simulink model "Attitude_control_RW_20b"  (R2022a)
settings: Solver=VariableStepAuto  StartTime=0.0  StopTime=100  FixedStep=0.0001  RelTol=1e-3
values from neighbouring files (symbols this model uses):
  D = 9.4e-5*Kt    (= 4.7e-06)    [motor_parameter.m]
  J = 1.94e-4*Kt    (= 9.7e-06)    [motor_parameter.m]
  kii = (J*(-Kt^2+kpo*R)*wn^2)/(Kt*(D^2+kpo^2+J^2*wn^2-2*J*kpo*wn*zeta+2*D*(kpo-J*wn*zeta)))    (= 0.394297267374)    [motor_parameter.m]
  kpi = -(D^2*R+J^2*R*wn^2+kpo*(Kt^2-2*J*R*wn*zeta)+D*(Kt^2+R*(kpo-2*J*wn*zeta))/(Kt*(D^2+kpo^2+J^2*wn^2-2*J*kpo*wn*zeta+2*D*(kpo-J*wn*zeta))))    (= 0.0794485412984)    [motor_parameter.m]
  kpo = 10    [motor_parameter.m]
  Kt = 0.05    [motor_parameter.m]
  L = 0.001    [motor_parameter.m]
  R = 14.3    [motor_parameter.m]
  Tc = 0.053*Kt    (= 0.00265)    [motor_parameter.m]
undefined symbols (not defined in the file or in its folder): b, Is, kk, Km, Q, q_init, Rgyro, Rstr, rw_Inertia, rw_SensorToBody, Ts, unit7, w0, w_dot_init, w_init, wRW_init
libraries: simulink_extras x13, sharedtransform x12, simulink x5, slpidlib x3, aerolibutil x2, sharedTrackingLibrary x1
(part 1 of 2)
settings Model: Creator=sokserey  LastModifiedBy=LabPC
settings SolverCC: ZeroCrossAlgorithm=Adaptive  AlgebraicLoopSolver=TrustRegion
settings DebuggingCC: IgnoredZcDiagnostic=none  UnconnectedInputMsg=warning  UnconnectedOutputMsg=warning  UnconnectedLineMsg=warning
settings RTWCC: DLArmComputeVersion=19.05

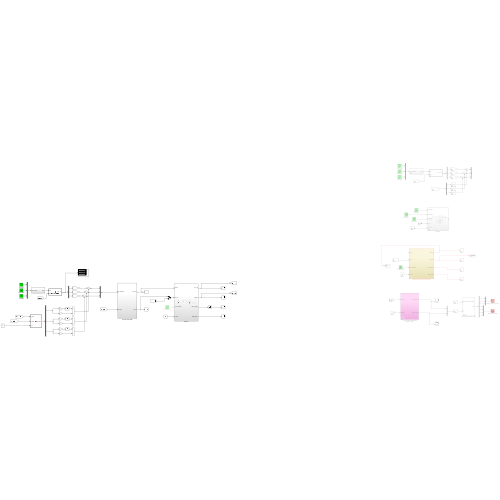
[thumbnail: Simulink's stored preview of the top-level diagram]
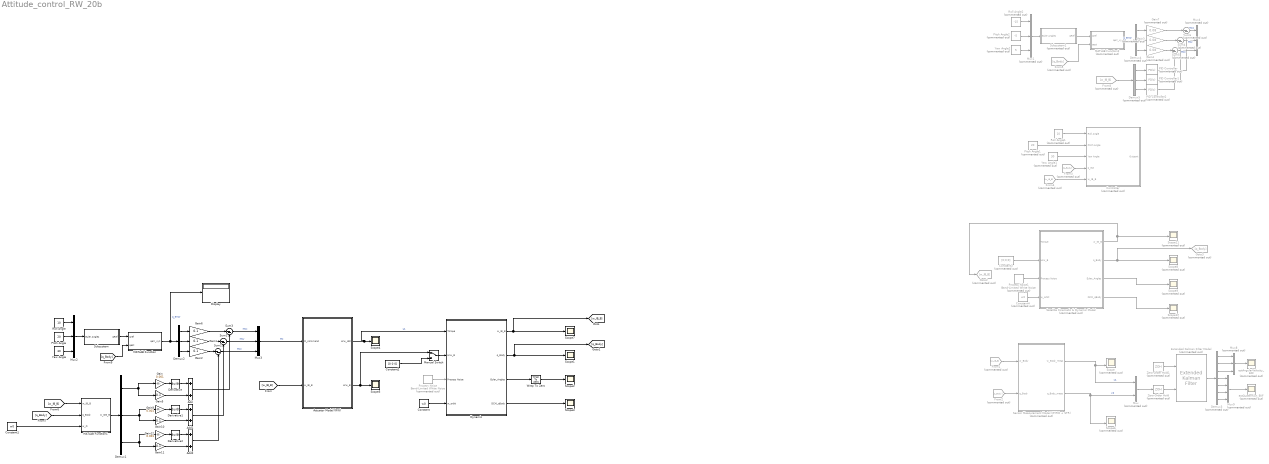
== system Attitude_control_RW_20b ==
  Actuator Model (RW) : Subsystem
  Add : Sum
  Add1 : Sum
  Add2 : Sum
  Constant : Constant  Value=w0
  Constant1 : Constant  Value=w0
  Constant2 : Constant  Value=[0 0 0]
  Constant3 : Constant  Commented=on  Value=[0;0;0]
  Constant4 : Constant  Commented=on  Value=w0
  Controller : Subsystem  Commented=on
  Demux1 : Demux  Outputs=3
  Demux2 : Demux  Outputs=3
  Demux3 : Demux  Commented=on  Outputs=7
  Demux4 : Demux  Commented=on  Outputs=3
  Demux5 : Demux  Commented=on  Outputs=3
  Derivative : Derivative
  Derivative1 : Derivative
  Derivative2 : Derivative
  Display : Display
  Dynamic : Subsystem
  "Extended Kalman Filter Model " : sharedTrackingLibrary/Extended Kalman Filter  Commented=on  StateTransitionFcn=dynamicFunctions2  HasStateTransitionJacobianFcn=off  HasAdditiveProcessNoise=Additive  ProcessNoise=diag(unit7)*Q  HasTimeVaryingProcessNoise=off  HasStateTransitionFcnExtraArgument=1  InitialState=[w_init; q_init]  InitialStateCovariance=1e-6  MeasurementFcn1=measurementFunction2  HasMeasurementJacobianFcn1=off  HasMeasurementEnablePort1=off  HasAdditiveMeasurementNoise1=Additive  MeasurementNoise1=Rconf4  HasTimeVaryingMeasurementNoise1=off  HasMeasurementFcnExtraArgument1=0  HasMeasurementWrapping1=off  MeasurementFcn2=myMeasurementFcn  HasMeasurementJacobianFcn2=off  HasMeasurementEnablePort2=off  HasAdditiveMeasurementNoise2=Additive  MeasurementNoise2=1  HasTimeVaryingMeasurementNoise2=off  HasMeasurementFcnExtraArgument2=0  HasMeasurementWrapping2=off  MeasurementFcn3=myMeasurementFcn  HasMeasurementJacobianFcn3=off  HasMeasurementEnablePort3=off  HasAdditiveMeasurementNoise3=Additive  MeasurementNoise3=1  HasTimeVaryingMeasurementNoise3=off  HasMeasurementFcnExtraArgument3=0  HasMeasurementWrapping3=off  MeasurementFcn4=myMeasurementFcn  HasMeasurementJacobianFcn4=off  HasMeasurementEnablePort4=off  HasAdditiveMeasurementNoise4=Additive  MeasurementNoise4=1  HasTimeVaryingMeasurementNoise4=off  HasMeasurementFcnExtraArgument4=0  HasMeasurementWrapping4=off  MeasurementFcn5=myMeasurementFcn  HasMeasurementJacobianFcn5=off  HasMeasurementEnablePort5=off  HasAdditiveMeasurementNoise5=Additive  MeasurementNoise5=1  HasTimeVaryingMeasurementNoise5=off  HasMeasurementFcnExtraArgument5=0  HasMeasurementWrapping5=off  EnableMultirate=off  StateTransitionFcnSampleTime=1  MeasurementFcn1SampleTime=1  MeasurementFcn2SampleTime=1  MeasurementFcn3SampleTime=1  MeasurementFcn4SampleTime=1  MeasurementFcn5SampleTime=1  UseCurrentEstimator=on  OutputStateCovariance=off  DataType=double  SampleTime=Ts  NumberOfMeasurements=1
      settings: SourceProductBaseCode=TF,AE,PW,CT,DR,ID,LP,NV,AR,RO,RR,UV,VE
  From1 : From  Commented=on  GotoTag=w_IB_B
  From2 : From  Commented=on  GotoTag=q_Body
  From3 : From  Commented=on  GotoTag=q_Body
  From4 : From  Commented=on  GotoTag=w_IB_B
  From5 : From  Commented=on  GotoTag=q_Body
  From8 : From  Commented=on  GotoTag=w_IB_B
  Gain : Gain  Gain=0.001
  Gain{1..2,5..6,10..11} (6 alike) : Gain  Gain=0.1
  Gain12 : Gain  Gain=0.001
  Gain3 : Gain  Commented=on  Gain=0.08
  Gain4 : Gain  Commented=on  Gain=0.08
  Gain7 : Gain  Commented=on  Gain=0.08
  Gain9 : Gain  Gain=0.001
  Goto2 : Goto  Commented=on  GotoTag=w_IB_B
  Goto3 : Goto  Commented=on  GotoTag=q_Body
  MATLAB Function : MATLAB Function  TreatAsAtomicUnit=on
  MATLAB Function1 : MATLAB Function  TreatAsAtomicUnit=on
  MATLAB Function2 : MATLAB Function  Commented=on  TreatAsAtomicUnit=on
  Manual Switch : ManualSwitch
  Mux : Mux  Commented=on  Inputs=2
  Mux1 : Mux  Commented=on  Inputs=3
  Mux2 : Mux  Inputs=3
  Mux3 : Mux  Inputs=3
  Mux4 : Mux  Commented=on  Inputs=3
  Mux8 : Mux  Commented=on  Inputs=3
  Mux9 : Mux  Commented=on
  PID Controller : slpidlib/PID Controller  Commented=on  Controller=PD  Form=Parallel  TimeDomain=Continuous-time  UseExternalTs=off  SampleTime=-1  IntegratorMethod=Forward Euler  FilterMethod=Forward Euler  ControllerParametersSource=internal  P=1  I=2  UseKiTs=off  D=2  N=100  UseFilter=on  TunerSelectOption=Transfer Function Based (PID Tuner App)  InitialConditionSource=internal  InitialConditionForIntegrator=0  InitialConditionForFilter=0  DifferentiatorICPrevScaledInput=0  ExternalReset=none  TrackingMode=off  Kt=1  LimitOutput=off  SatLimitsSource=internal  UpperSaturationLimit=inf  LowerSaturationLimit=-inf  LinearizeAsGain=on  AntiWindupMode=none  Kb=1  POutMin=[]  POutMax=[]  IOutMin=[]  IOutMax=[]  DOutMin=[]  DOutMax=[]  NOutMin=[]  NOutMax=[]  SumOutMin=[]  SumOutMax=[]  SaturationOutMin=[]  SaturationOutMax=[]  PParamMin=[]  PParamMax=[]  IParamMin=[]  IParamMax=[]  DParamMin=[]  DParamMax=[]  NParamMin=[]  NParamMax=[]  KbParamMin=[]  KbParamMax=[]  KtParamMin=[]  KtParamMax=[]  KbOutMin=[]  KbOutMax=[]  KtOutMin=[]  KtOutMax=[]  IntegratorOutMin=[]  IntegratorOutMax=[]  FilterOutMin=[]  FilterOutMax=[]  SumI1OutMin=[]  SumI1OutMax=[]  SumI2OutMin=[]  SumI2OutMax=[]  SumI3OutMin=[]  SumI3OutMax=[]  SumI4OutMin=[]  SumI4OutMax=[]  SumDOutMin=[]  SumDOutMax=[]  DifferentiatorOutMin=[]  DifferentiatorOutMax=[]  FilterDiffOutCoefMin=[]  FilterDiffOutCoefMax=[]  ReciprocalOutMin=[]  ReciprocalOutMax=[]  SumDenOutMin=[]  SumDenOutMax=[]  SumNumOutMin=[]  SumNumOutMax=[]  DivideOutMin=[]  DivideOutMax=[]  UdiffTsProdOutMin=[]  UdiffTsProdOutMax=[]  NTsProdOutMin=[]  NTsProdOutMax=[]  UintegralTsProdOutMin=[]  UintegralTsProdOutMax=[]  UngainTsProdOutMin=[]  UngainTsProdOutMax=[]  IntegratorContinuousStateAttributes=''  IntegratorStateMustResolveToSignalObject=off  IntegratorRTWStateStorageClass=Auto  FilterContinuousStateAttributes=''  FilterStateMustResolveToSignalObject=off  FilterRTWStateStorageClass=Auto  ParallelPVariant=InternalParameters  IdealPVariant=Disabled  IVariant=Disabled  DVariant=InternalParameters  IntegratorVariant=Disabled  SatVariant=Disabled  AWVariant=Disabled  PCopyVariant=Disabled  TRVariant=Disabled  FdbkBlocksVariant=Forward  IdealPFdbkVariant=Disabled  SatFdbkVariant=Disabled  DerivativeFilterVariant=ContFilter  NVariant=InternalParameters  NCopyVariant=Disabled  FilterICVariant=InternalICsFilter  IntegratorICVariant=Disabled  ExternalResetVariant=Disabled  TRSumVariant=Passthrough  SumFdbkVariant=Disabled  SumVariant=Sum_PD  TsampFilterVariant=InternalTs  TsampNgainVariant=Passthrough  TsampIntegralVariant=Disabled_SignalSpec  ExternalSaturationOutDataTypeStr=Inherit: Same as second input  aMode=0
  PID Controller1 : slpidlib/PID Controller  Commented=on  Controller=PD  Form=Parallel  TimeDomain=Continuous-time  UseExternalTs=off  SampleTime=-1  IntegratorMethod=Forward Euler  FilterMethod=Forward Euler  ControllerParametersSource=internal  P=1  I=2  UseKiTs=off  D=2  N=100  UseFilter=on  TunerSelectOption=Transfer Function Based (PID Tuner App)  InitialConditionSource=internal  InitialConditionForIntegrator=0  InitialConditionForFilter=0  DifferentiatorICPrevScaledInput=0  ExternalReset=none  TrackingMode=off  Kt=1  LimitOutput=off  SatLimitsSource=internal  UpperSaturationLimit=inf  LowerSaturationLimit=-inf  LinearizeAsGain=on  AntiWindupMode=none  Kb=1  POutMin=[]  POutMax=[]  IOutMin=[]  IOutMax=[]  DOutMin=[]  DOutMax=[]  NOutMin=[]  NOutMax=[]  SumOutMin=[]  SumOutMax=[]  SaturationOutMin=[]  SaturationOutMax=[]  PParamMin=[]  PParamMax=[]  IParamMin=[]  IParamMax=[]  DParamMin=[]  DParamMax=[]  NParamMin=[]  NParamMax=[]  KbParamMin=[]  KbParamMax=[]  KtParamMin=[]  KtParamMax=[]  KbOutMin=[]  KbOutMax=[]  KtOutMin=[]  KtOutMax=[]  IntegratorOutMin=[]  IntegratorOutMax=[]  FilterOutMin=[]  FilterOutMax=[]  SumI1OutMin=[]  SumI1OutMax=[]  SumI2OutMin=[]  SumI2OutMax=[]  SumI3OutMin=[]  SumI3OutMax=[]  SumI4OutMin=[]  SumI4OutMax=[]  SumDOutMin=[]  SumDOutMax=[]  DifferentiatorOutMin=[]  DifferentiatorOutMax=[]  FilterDiffOutCoefMin=[]  FilterDiffOutCoefMax=[]  ReciprocalOutMin=[]  ReciprocalOutMax=[]  SumDenOutMin=[]  SumDenOutMax=[]  SumNumOutMin=[]  SumNumOutMax=[]  DivideOutMin=[]  DivideOutMax=[]  UdiffTsProdOutMin=[]  UdiffTsProdOutMax=[]  NTsProdOutMin=[]  NTsProdOutMax=[]  UintegralTsProdOutMin=[]  UintegralTsProdOutMax=[]  UngainTsProdOutMin=[]  UngainTsProdOutMax=[]  IntegratorContinuousStateAttributes=''  IntegratorStateMustResolveToSignalObject=off  IntegratorRTWStateStorageClass=Auto  FilterContinuousStateAttributes=''  FilterStateMustResolveToSignalObject=off  FilterRTWStateStorageClass=Auto  ParallelPVariant=InternalParameters  IdealPVariant=Disabled  IVariant=Disabled  DVariant=InternalParameters  IntegratorVariant=Disabled  SatVariant=Disabled  AWVariant=Disabled  PCopyVariant=Disabled  TRVariant=Disabled  FdbkBlocksVariant=Forward  IdealPFdbkVariant=Disabled  SatFdbkVariant=Disabled  DerivativeFilterVariant=ContFilter  NVariant=InternalParameters  NCopyVariant=Disabled  FilterICVariant=InternalICsFilter  IntegratorICVariant=Disabled  ExternalResetVariant=Disabled  TRSumVariant=Passthrough  SumFdbkVariant=Disabled  SumVariant=Sum_PD  TsampFilterVariant=InternalTs  TsampNgainVariant=Passthrough  TsampIntegralVariant=Disabled_SignalSpec  ExternalSaturationOutDataTypeStr=Inherit: Same as second input  aMode=0
  PID Controller2 : slpidlib/PID Controller  Commented=on  Controller=PD  Form=Parallel  TimeDomain=Continuous-time  UseExternalTs=off  SampleTime=-1  IntegratorMethod=Forward Euler  FilterMethod=Forward Euler  ControllerParametersSource=internal  P=1  I=2  UseKiTs=off  D=2  N=100  UseFilter=on  TunerSelectOption=Transfer Function Based (PID Tuner App)  InitialConditionSource=internal  InitialConditionForIntegrator=0  InitialConditionForFilter=0  DifferentiatorICPrevScaledInput=0  ExternalReset=none  TrackingMode=off  Kt=1  LimitOutput=off  SatLimitsSource=internal  UpperSaturationLimit=inf  LowerSaturationLimit=-inf  LinearizeAsGain=on  AntiWindupMode=none  Kb=1  POutMin=[]  POutMax=[]  IOutMin=[]  IOutMax=[]  DOutMin=[]  DOutMax=[]  NOutMin=[]  NOutMax=[]  SumOutMin=[]  SumOutMax=[]  SaturationOutMin=[]  SaturationOutMax=[]  PParamMin=[]  PParamMax=[]  IParamMin=[]  IParamMax=[]  DParamMin=[]  DParamMax=[]  NParamMin=[]  NParamMax=[]  KbParamMin=[]  KbParamMax=[]  KtParamMin=[]  KtParamMax=[]  KbOutMin=[]  KbOutMax=[]  KtOutMin=[]  KtOutMax=[]  IntegratorOutMin=[]  IntegratorOutMax=[]  FilterOutMin=[]  FilterOutMax=[]  SumI1OutMin=[]  SumI1OutMax=[]  SumI2OutMin=[]  SumI2OutMax=[]  SumI3OutMin=[]  SumI3OutMax=[]  SumI4OutMin=[]  SumI4OutMax=[]  SumDOutMin=[]  SumDOutMax=[]  DifferentiatorOutMin=[]  DifferentiatorOutMax=[]  FilterDiffOutCoefMin=[]  FilterDiffOutCoefMax=[]  ReciprocalOutMin=[]  ReciprocalOutMax=[]  SumDenOutMin=[]  SumDenOutMax=[]  SumNumOutMin=[]  SumNumOutMax=[]  DivideOutMin=[]  DivideOutMax=[]  UdiffTsProdOutMin=[]  UdiffTsProdOutMax=[]  NTsProdOutMin=[]  NTsProdOutMax=[]  UintegralTsProdOutMin=[]  UintegralTsProdOutMax=[]  UngainTsProdOutMin=[]  UngainTsProdOutMax=[]  IntegratorContinuousStateAttributes=''  IntegratorStateMustResolveToSignalObject=off  IntegratorRTWStateStorageClass=Auto  FilterContinuousStateAttributes=''  FilterStateMustResolveToSignalObject=off  FilterRTWStateStorageClass=Auto  ParallelPVariant=InternalParameters  IdealPVariant=Disabled  IVariant=Disabled  DVariant=InternalParameters  IntegratorVariant=Disabled  SatVariant=Disabled  AWVariant=Disabled  PCopyVariant=Disabled  TRVariant=Disabled  FdbkBlocksVariant=Forward  IdealPFdbkVariant=Disabled  SatFdbkVariant=Disabled  DerivativeFilterVariant=ContFilter  NVariant=InternalParameters  NCopyVariant=Disabled  FilterICVariant=InternalICsFilter  IntegratorICVariant=Disabled  ExternalResetVariant=Disabled  TRSumVariant=Passthrough  SumFdbkVariant=Disabled  SumVariant=Sum_PD  TsampFilterVariant=InternalTs  TsampNgainVariant=Passthrough  TsampIntegralVariant=Disabled_SignalSpec  ExternalSaturationOutDataTypeStr=Inherit: Same as second input  aMode=0
  Pitch Angle : Constant  Value=20
  Pitch Angle1 : Constant  Commented=on  Value=20
  Pitch Angle2 : Constant  Commented=on  Value=-5
  Process Noise : simulink/Sources/Band-Limited White Noise  Commented=on  Cov=Q*Ts  Ts=Ts  seed=[23341]
  Process Noise1 : simulink/Sources/Band-Limited White Noise  Commented=on  Cov=Q*Ts  Ts=Ts  seed=[23341]
  Roll Angle : Constant  Value=10
  Roll Angle1 : Constant  Commented=on  Value=10
  Roll Angle2 : Constant  Commented=on  Value=-15
  Satellite Kinematic & Dynamic Model : Subsystem  Commented=on
  Scope : Scope  Commented=on  NumInputPorts=2
  Scope{1..5,7} (6 alike) : Scope
  Scope{8..11} (4 alike) : Scope  Commented=on
  Scope6 : Scope  Commented=on  NumInputPorts=2
  Sensor Measurement Model (GYRO + STR) : Subsystem  Commented=on
  Subsystem : Subsystem
  Subsystem1 : Subsystem  Commented=on
  Sum1 : Sum  Inputs=|--
  Sum2 : Sum  Inputs=|--
  Sum3 : Sum  Inputs=|--
  Sum4 : Sum  Commented=on  Inputs=|--
  Sum5 : Sum  Commented=on  Inputs=|--
  Sum6 : Sum  Commented=on  Inputs=|--
  Wrap To Zero : simulink/Discontinuities/Wrap To Zero  Threshold=360
      settings: SourceProductBaseCode=SL
  Yaw Angle : Constant  Value=30
  Yaw Angle1 : Constant  Commented=on  Value=30
  Yaw Angle2 : Constant  Commented=on  Value=5
  Zero-Order Hold : ZeroOrderHold  Commented=on  SampleTime=Ts
  Zero-Order Hold1 : ZeroOrderHold  Commented=on  SampleTime=Ts
  estAngularVelocity_EKF : Scope  Commented=on
  "estQuaternion_EKF " : Scope  Commented=on
  wires:
  Process Noise/1 -> Dynamic/3("Process Noise ")
  Constant/1 -> Dynamic/4(w_orbit)
  Dynamic/2(q_Body) -> [q_Body], Scope1/1
  Dynamic/3(Euler_Angles) -> Wrap To Zero/1
  Dynamic/4(DCM_qBody) -> Scope3/1
  Zero-Order Hold1/1 -> "Extended Kalman Filter Model "/1
  Demux3/2 -> Mux8/2
  Demux3/3 -> Mux8/3
  Demux3/6 -> Mux9/3
  Demux3/4 -> Mux9/1
  Mux9/1 -> "estQuaternion_EKF "/1
  Demux3/5 -> Mux9/2
  "Extended Kalman Filter Model "/1 -> Demux3/1
  Demux3/1 -> Mux8/1
  Zero-Order Hold/1 -> "Extended Kalman Filter Model "/2
  [w_IB_B] -> Actuator Model (RW)/2(w_IB_B)
  Actuator Model (RW)/1("Hrw_dot ") -> Dynamic/1(Torque), Scope4/1  "u1"
  From1/1 -> Sensor Measurement Model (GYRO + STR)/1(w_Body)
  Sensor Measurement Model (GYRO + STR)/1(w_Body_meas) -> Mux/1, Scope/2  "y1"
  From2/1 -> Sensor Measurement Model (GYRO + STR)/2(q_Body)
  Sensor Measurement Model (GYRO + STR)/2(q_Body_meas) -> Scope6/2, Mux/2  "y2"
  Mux/1 -> Zero-Order Hold/1
  Roll Angle/1 -> Mux2/1
  Sum1/1 -> Mux3/2  "Mcy"
  MATLAB Function/1(qerr_xyz) -> Display/1, Demux2/1  "q_error"
  Sum3/1 -> Mux3/1  "Mcx"
  Gain2/1 -> Sum2/1
  Sum2/1 -> Mux3/3  "Mcz"
  Demux2/2 -> Gain1/1
  Demux2/1 -> Gain6/1
  Gain6/1 -> Sum3/1
  Yaw Angle/1 -> Mux2/3
  Subsystem/1(qRef) -> MATLAB Function/1(qref)
  Gain1/1 -> Sum1/1
  Pitch Angle/1 -> Mux2/2
  Mux2/1 -> Subsystem/1(Euler Angles)
  Demux2/3 -> Gain2/1
  Mux8/1 -> estAngularVelocity_EKF/1
  Demux3/7 -> Mux9/4
  Dynamic/1(w_IB_B) -> [w_IB_B], Scope7/1
  Roll Angle1/1 -> Controller/1("Roll Angle ")
  Pitch Angle1/1 -> Controller/2("Pitch Angle ")
  Yaw Angle1/1 -> Controller/3("Yaw Angle ")
  Actuator Model (RW)/2(Hrw_B) -> Manual Switch/1, Scope5/1
  From3/1 -> Controller/4(q_est)
  From4/1 -> Controller/5(w_IB_B)
  Derivative/1 -> Add/1
  Gain5/1 -> Add/2
  Gain9/1 -> Derivative1/1
  Gain10/1 -> Add1/2
  Gain11/1 -> Add2/2
  Derivative1/1 -> Add1/1
  Demux1/3 -> Gain12/1, Gain11/1
  Gain/1 -> Derivative/1
  Derivative2/1 -> Add2/1
  Demux1/1 -> Gain/1, Gain5/1
  Demux1/2 -> Gain9/1, Gain10/1
  Gain12/1 -> Derivative2/1
  [w_IB_B] -> MATLAB Function1/1(w_IB_B)
  [q_Body] -> MATLAB Function1/2(q_Body)
  Constant1/1 -> MATLAB Function1/3(w_O)
  MATLAB Function1/1(w_OB_B) -> Demux1/1
  Manual Switch/1 -> Dynamic/2(Hrw_B)
  Constant2/1 -> Manual Switch/2
  Demux4/2 -> Gain3/1
  Sum6/1 -> Mux4/1  "Mcx"
  Sum5/1 -> Mux4/3  "Mcz"
  Gain7/1 -> Sum6/1
  PID Controller1/1 -> Sum4/2
  PID Controller2/1 -> Sum5/2
  Gain4/1 -> Sum5/1
  Sum4/1 -> Mux4/2  "Mcy"
  Demux5/3 -> PID Controller2/1
  PID Controller/1 -> Sum6/2
  Subsystem1/1(qRef) -> MATLAB Function2/1(qref)
  Demux5/1 -> PID Controller/1
  Demux5/2 -> PID Controller1/1
  Demux4/3 -> Gain4/1
  MATLAB Function2/1(qerr_xyz) -> Demux4/1  "q_error"
  Demux4/1 -> Gain7/1
  Pitch Angle2/1 -> Mux1/2
  Gain3/1 -> Sum4/1
  Yaw Angle2/1 -> Mux1/3
  Roll Angle2/1 -> Mux1/1
  Mux1/1 -> Subsystem1/1(Euler Angles)
  From8/1 -> Demux5/1
  From5/1 -> MATLAB Function2/2(qest)
  Constant3/1 -> Satellite Kinematic & Dynamic Model/2(Hrw_B)
  Process Noise1/1 -> Satellite Kinematic & Dynamic Model/3("Process Noise ")
  Constant4/1 -> Satellite Kinematic & Dynamic Model/4(w_orbit)
  Satellite Kinematic & Dynamic Model/1(w_IB_B) -> Scope11/1, Goto2/1
  Satellite Kinematic & Dynamic Model/4(DCM_qBody) -> Scope10/1
  Satellite Kinematic & Dynamic Model/3(Euler_Angles) -> Scope9/1
  Satellite Kinematic & Dynamic Model/2(q_Body) -> Scope8/1, Goto3/1
  Add/1 -> Sum3/2
  Add1/1 -> Sum1/2
  Add2/1 -> Sum2/2
  [q_Body] -> MATLAB Function/2(qest)
  Mux3/1 -> Actuator Model (RW)/1("M_command ")  "Mc"
  Wrap To Zero/1 -> Scope2/1

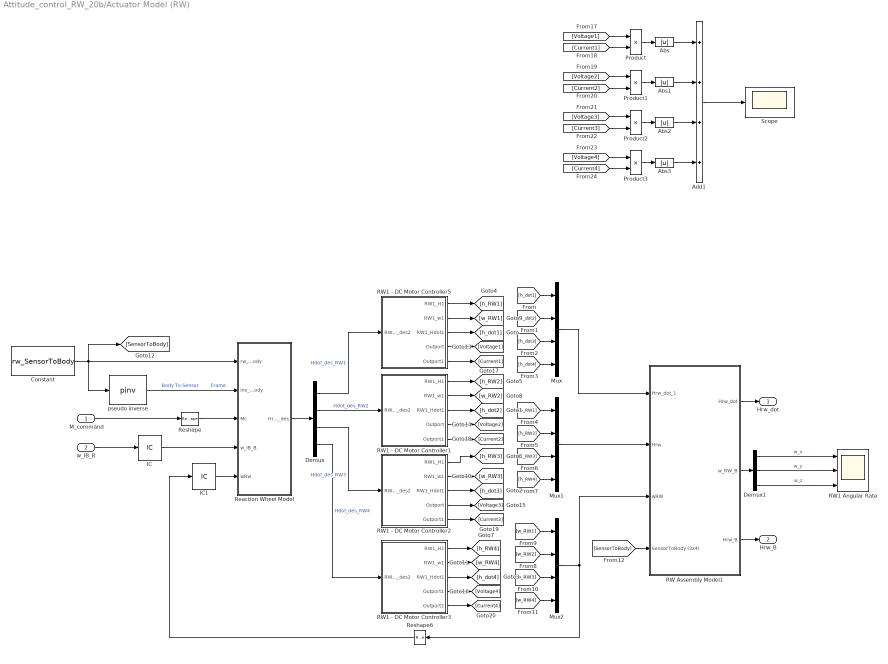
== system Attitude_control_RW_20b/Actuator Model (RW) ==
  "M_command " : Inport
  w_IB_B : Inport  Port=2
  Abs{,1..3} (4 alike) : Abs  SaturateOnIntegerOverflow=off
  Add1 : Sum  Inputs=++++
  Constant : Constant  Value=rw_SensorToBody
  Demux : Demux
  Demux1 : Demux  Outputs=3
  IC : InitialCondition  Value=w_init
  IC1 : InitialCondition  Value=wRW_init
  Mux : Mux
  Mux1 : Mux
  Mux2 : Mux
  Product{,1..3} (4 alike) : Product
  RW Assembly Model1 : Subsystem
  RW1 - DC Motor Controller1 : Subsystem
  RW1 - DC Motor Controller2 : Subsystem
  RW1 - DC Motor Controller3 : Subsystem
  RW1 - DC Motor Controller5 : Subsystem
  RW1 Angular Rate : Scope  NumInputPorts=3
  Reaction Wheel Model : MATLAB Function  TreatAsAtomicUnit=on
  Reshape : Reshape  OutputDimensionality=Column vector (2-D)
  Reshape6 : Reshape  OutputDimensionality=Column vector (2-D)
  Scope : Scope
  pseudo inverse : MATLABFcn  MATLABFcn=pinv  Output1D=off
  "Hrw_dot " : Outport  VectorParamsAs1DForOutWhenUnconnected=off
  Hrw_B : Outport  Port=2  VectorParamsAs1DForOutWhenUnconnected=off
  wires:
  Demux1/3 -> RW1 Angular Rate/3  "w_z"
  Demux1/1 -> RW1 Angular Rate/1  "w_x"
  Demux1/2 -> RW1 Angular Rate/2  "w_y"
  "M_command "/1 -> Reshape/1
  Reaction Wheel Model/1(Hrw_dot_des) -> Demux/1
  [h_dot1] -> Mux/1
  [h_dot2] -> Mux/2
  [h_dot3] -> Mux/3
  [h_dot4] -> Mux/4
  Mux/1 -> RW Assembly Model1/1(Hrw_dot_1)
  [h_RW1] -> Mux1/1
  [h_RW2] -> Mux1/2
  [h_RW3] -> Mux1/3
  [h_RW4] -> Mux1/4
  Mux1/1 -> RW Assembly Model1/2(Hrw)
  [w_RW2] -> Mux2/2
  [w_RW1] -> Mux2/1
  [w_RW3] -> Mux2/3
  [w_RW4] -> Mux2/4
  pseudo inverse/1 -> Reaction Wheel Model/2(inv_rwSensorToBody)  "Body To Sensor         Frame"
  Reshape/1 -> Reaction Wheel Model/3(Mc)
  Constant/1 -> pseudo inverse/1, [SensorToBody], Reaction Wheel Model/1(rw_SensorToBody)
  [SensorToBody] -> RW Assembly Model1/4(SensorToBody (3x4))
  RW Assembly Model1/2(w_RW_B) -> Demux1/1
  RW Assembly Model1/1(Hrw_dot) -> "Hrw_dot "/1
  Mux2/1 -> Reshape6/1, RW Assembly Model1/3(wRW)
  Reshape6/1 -> IC1/1
  w_IB_B/1 -> IC/1
  IC/1 -> Reaction Wheel Model/4(w_IB_B)
  IC1/1 -> Reaction Wheel Model/5(wRw)
  RW Assembly Model1/3(Hrw_B) -> Hrw_B/1
  Demux/1 -> RW1 - DC Motor Controller5/1(RW1_Hdot_des2)  "Hdot_des_RW1"
  Demux/2 -> RW1 - DC Motor Controller1/1(RW1_Hdot_des2)  "Hdot_des_RW2"
  Demux/3 -> RW1 - DC Motor Controller2/1(RW1_Hdot_des2)  "Hdot_des_RW3"
  Demux/4 -> RW1 - DC Motor Controller3/1(RW1_Hdot_des2)  "Hdot_des_RW4"
  RW1 - DC Motor Controller5/1(RW1_H1) -> [h_RW1]
  RW1 - DC Motor Controller5/2(RW1_w1) -> [w_RW1]
  RW1 - DC Motor Controller5/3(RW1_Hdot1) -> [h_dot1]
  RW1 - DC Motor Controller1/1(RW1_H1) -> [h_RW2]
  RW1 - DC Motor Controller1/2(RW1_w1) -> [w_RW2]
  RW1 - DC Motor Controller1/3(RW1_Hdot1) -> [h_dot2]
  RW1 - DC Motor Controller2/1(RW1_H1) -> [h_RW3]
  RW1 - DC Motor Controller2/2(RW1_w1) -> [w_RW3]
  RW1 - DC Motor Controller2/3(RW1_Hdot1) -> [h_dot3]
  RW1 - DC Motor Controller3/1(RW1_H1) -> [h_RW4]
  RW1 - DC Motor Controller3/2(RW1_w1) -> [w_RW4]
  RW1 - DC Motor Controller3/3(RW1_Hdot1) -> [h_dot4]
  RW1 - DC Motor Controller5/4(Outport) -> [Voltage1]
  RW1 - DC Motor Controller1/4(Outport) -> [Voltage2]
  RW1 - DC Motor Controller2/4(Outport) -> [Voltage3]
  RW1 - DC Motor Controller3/4(Outport1) -> [Voltage4]
  RW1 - DC Motor Controller5/5(Outport1) -> [Current1]
  RW1 - DC Motor Controller1/5(Outport1) -> [Current2]
  RW1 - DC Motor Controller2/5(Outport1) -> [Current3]
  RW1 - DC Motor Controller3/5(Outport2) -> [Current4]
  [Voltage1] -> Product/1
  [Current1] -> Product/2
  Product/1 -> Abs/1
  Product1/1 -> Abs1/1
  [Current2] -> Product1/2
  [Voltage2] -> Product1/1
  [Voltage3] -> Product2/1
  [Current3] -> Product2/2
  Product2/1 -> Abs2/1
  Product3/1 -> Abs3/1
  [Current4] -> Product3/2
  [Voltage4] -> Product3/1
  Abs/1 -> Add1/1
  Abs1/1 -> Add1/2
  Abs2/1 -> Add1/3
  Abs3/1 -> Add1/4
  Add1/1 -> Scope/1

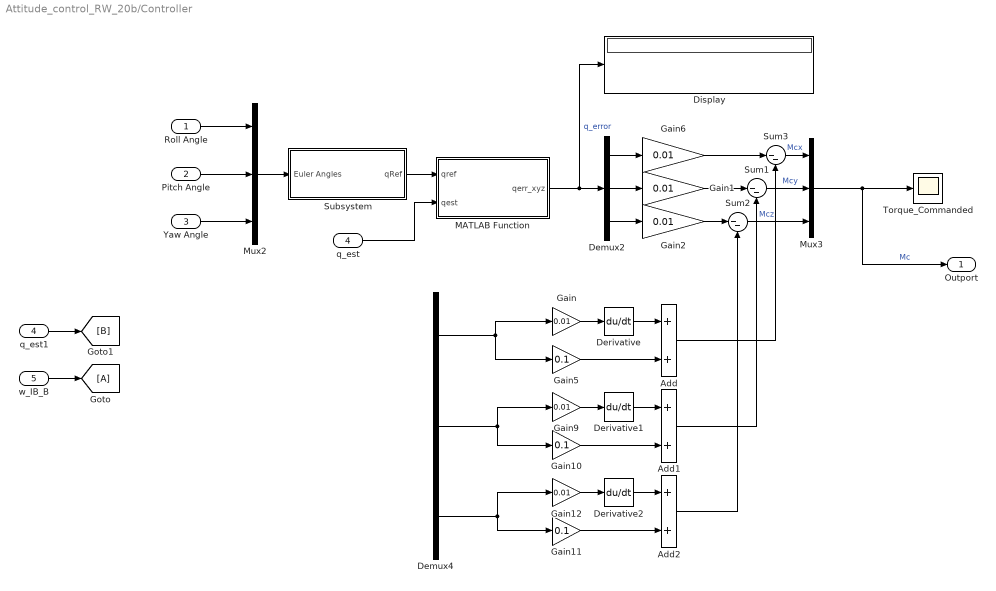
== system Attitude_control_RW_20b/Controller ==
  "Roll Angle " : Inport
  "Pitch Angle " : Inport  Port=2
  "Yaw Angle " : Inport  Port=3
  q_est : Inport  Port=4
  w_IB_B : Inport  Port=5
  Add : Sum
  Add1 : Sum
  Add2 : Sum
  Demux2 : Demux  Outputs=3
  Demux4 : Demux  Outputs=3
  Derivative : Derivative
  Derivative1 : Derivative
  Derivative2 : Derivative
  Display : Display
  Gain{,1..2,6,9,12} (6 alike) : Gain  Gain=0.01
  Gain10 : Gain  Gain=0.1
  Gain11 : Gain  Gain=0.1
  Gain5 : Gain  Gain=0.1
  Goto : Goto
  MATLAB Function : MATLAB Function  TreatAsAtomicUnit=on
  Mux2 : Mux  Inputs=3
  Mux3 : Mux  Inputs=3
  Subsystem : Subsystem
  Sum1 : Sum  Inputs=|--
  Sum2 : Sum  Inputs=|--
  Sum3 : Sum  Inputs=|--
  Torque_Commanded : Scope
  q_est1 : InportShadow  Port=4
  Outport : Outport
  wires:
  Mux2/1 -> Subsystem/1(Euler Angles)
  MATLAB Function/1(qerr_xyz) -> Display/1, Demux2/1  "q_error"
  Sum2/1 -> Mux3/3  "Mcz"
  Demux2/3 -> Gain2/1
  Sum3/1 -> Mux3/1  "Mcx"
  Mux3/1 -> Outport/1, Torque_Commanded/1  "Mc"
  Gain1/1 -> Sum1/1
  Subsystem/1(qRef) -> MATLAB Function/1(qref)
  Sum1/1 -> Mux3/2  "Mcy"
  Gain6/1 -> Sum3/1
  Gain2/1 -> Sum2/1
  Demux2/2 -> Gain1/1
  Demux2/1 -> Gain6/1
  "Roll Angle "/1 -> Mux2/1
  "Pitch Angle "/1 -> Mux2/2
  "Yaw Angle "/1 -> Mux2/3
  Gain5/1 -> Add/2
  Gain/1 -> Derivative/1
  Derivative/1 -> Add/1
  Derivative1/1 -> Add1/1
  Gain9/1 -> Derivative1/1
  Gain10/1 -> Add1/2
  Gain11/1 -> Add2/2
  Gain12/1 -> Derivative2/1
  Derivative2/1 -> Add2/1
  Demux4/1 -> Gain/1, Gain5/1
  Demux4/2 -> Gain9/1, Gain10/1
  Demux4/3 -> Gain12/1, Gain11/1
  Add/1 -> Sum3/2
  Add1/1 -> Sum1/2
  Add2/1 -> Sum2/2
  q_est/1 -> MATLAB Function/2(qest)
  w_IB_B/1 -> Goto/1
  q_est1/1 -> [B]

== system Attitude_control_RW_20b/Dynamic ==
  Torque : Inport
  Hrw_B : Inport  Port=2
  "Process Noise " : Inport  Port=3
  w_orbit : Inport  Port=4
  Display2 : Display
  Dynamic Model : Subsystem
  Kinematic Model1 : Subsystem
  Subsystem : Subsystem
  Subsystem1 : Subsystem
  Sum1 : Sum  Inputs=|++
  Sum2 : Sum  Inputs=|++
  Terminator : Terminator
  w_IB_B : Outport  VectorParamsAs1DForOutWhenUnconnected=off
  q_Body : Outport  Port=2  VectorParamsAs1DForOutWhenUnconnected=off
  Euler_Angles : Outport  Port=3  VectorParamsAs1DForOutWhenUnconnected=off
  DCM_qBody : Outport  Port=4  VectorParamsAs1DForOutWhenUnconnected=off
  wires:
  Sum2/1 -> Dynamic Model/2("Hrw_B ")
  Dynamic Model/1(w_IB_B) -> Kinematic Model1/1(w_IB_B), w_IB_B/1
  Hrw_B/1 -> Sum2/1
  Sum1/1 -> Dynamic Model/1(Mc+Md)
  Subsystem1/1(Euler Angle) -> Euler_Angles/1
  Torque/1 -> Sum1/1
  Kinematic Model1/2(w_OB_B) -> Terminator/1
  Kinematic Model1/1(qBody) -> Subsystem/1(qest), q_Body/1
  "Process Noise "/1 -> Sum2/2, Sum1/2
  Subsystem/1("DCM ") -> Subsystem1/1("DCM "), Display2/1, DCM_qBody/1
  w_orbit/1 -> Kinematic Model1/2(w_orbit)

== system Attitude_control_RW_20b/Satellite Kinematic & Dynamic Model ==
  Torque : Inport
  Hrw_B : Inport  Port=2
  "Process Noise " : Inport  Port=3
  w_orbit : Inport  Port=4
  Display2 : Display
  Dynamic Model : Subsystem
  Kinematic Model1 : Subsystem
  Subsystem : Subsystem
  Subsystem1 : Subsystem
  Sum1 : Sum  Inputs=|++
  Sum2 : Sum  Inputs=|++
  Terminator : Terminator
  w_IB_B : Outport  VectorParamsAs1DForOutWhenUnconnected=off
  q_Body : Outport  Port=2  VectorParamsAs1DForOutWhenUnconnected=off
  Euler_Angles : Outport  Port=3  VectorParamsAs1DForOutWhenUnconnected=off
  DCM_qBody : Outport  Port=4  VectorParamsAs1DForOutWhenUnconnected=off
  wires:
  Kinematic Model1/1(qBody) -> Subsystem/1(qest), q_Body/1
  w_orbit/1 -> Kinematic Model1/2(w_orbit)
  "Process Noise "/1 -> Sum2/2, Sum1/2
  Torque/1 -> Sum1/1
  Sum1/1 -> Dynamic Model/1(Mc+Md)
  Kinematic Model1/2(w_OB_B) -> Terminator/1
  Dynamic Model/1(w_IB_B) -> Kinematic Model1/1(w_IB_B), w_IB_B/1
  Subsystem/1("DCM ") -> Display2/1, DCM_qBody/1, Subsystem1/1("DCM ")
  Subsystem1/1(Euler Angle) -> Euler_Angles/1
  Hrw_B/1 -> Sum2/1
  Sum2/1 -> Dynamic Model/2("Hrw_B ")

== system Attitude_control_RW_20b/Sensor Measurement Model (GYRO + STR) ==
  w_Body : Inport
  q_Body : Inport  Port=2
  GYRO Sensor Model : Subsystem
  Normalization Model : Subsystem
  Star Tracker Model : Subsystem
  w_Body_meas : Outport  VectorParamsAs1DForOutWhenUnconnected=off
  q_Body_meas : Outport  Port=2  VectorParamsAs1DForOutWhenUnconnected=off
  wires:
  GYRO Sensor Model/1(w_Body_meas) -> w_Body_meas/1
  w_Body/1 -> GYRO Sensor Model/1(w_Body)
  q_Body/1 -> Star Tracker Model/1(q_Body)
  Normalization Model/1(Normalized_u) -> q_Body_meas/1
  Star Tracker Model/1(q_Body_meas) -> Normalization Model/1(u)

== system Attitude_control_RW_20b/Subsystem ==
  Euler Angles : Inport
  Degrees to Radians1 : simulink_extras/Transformations/Degrees to Radians
  Direction Cosine Matrix to Quaternions : sharedtransform/Direction Cosine Matrix  to Quaternions  aMode=0  action=None  tolerance=eps(2)
      settings: SourceProductBaseCode=AE,PW,DR,MT,VE
  Rotation Angles to Direction Cosine Matrix : sharedtransform/Rotation Angles to Direction Cosine Matrix  rotationOrder=ZYX  aMode=aMode
      settings: SourceProductBaseCode=AE,PW,DR,MT,VE
  Subsystem1 : Subsystem
  qRef : Outport  VectorParamsAs1DForOutWhenUnconnected=off
  wires:
  Euler Angles/1 -> Degrees to Radians1/1
  Degrees to Radians1/1 -> Rotation Angles to Direction Cosine Matrix/1
  Rotation Angles to Direction Cosine Matrix/1 -> Direction Cosine Matrix to Quaternions/1
  Direction Cosine Matrix to Quaternions/1 -> Subsystem1/1(q0,q1,q2,q3)
  Subsystem1/1(q1,q2,q3,q4) -> qRef/1

== system Attitude_control_RW_20b/Subsystem1 ==
  Euler Angles : Inport
  Degrees to Radians1 : simulink_extras/Transformations/Degrees to Radians
  Direction Cosine Matrix to Quaternions : sharedtransform/Direction Cosine Matrix  to Quaternions  aMode=0  action=None  tolerance=eps(2)
      settings: SourceProductBaseCode=AE,PW,DR,MT,VE
  Rotation Angles to Direction Cosine Matrix : sharedtransform/Rotation Angles to Direction Cosine Matrix  rotationOrder=ZYX  aMode=aMode
      settings: SourceProductBaseCode=AE,PW,DR,MT,VE
  Subsystem1 : Subsystem
  qRef : Outport  VectorParamsAs1DForOutWhenUnconnected=off
  wires:
  Euler Angles/1 -> Degrees to Radians1/1
  Degrees to Radians1/1 -> Rotation Angles to Direction Cosine Matrix/1
  Rotation Angles to Direction Cosine Matrix/1 -> Direction Cosine Matrix to Quaternions/1
  Direction Cosine Matrix to Quaternions/1 -> Subsystem1/1(q0,q1,q2,q3)
  Subsystem1/1(q1,q2,q3,q4) -> qRef/1

== system Attitude_control_RW_20b/Actuator Model (RW)/RW Assembly Model1 ==
  Hrw_dot_1 : Inport
  Hrw : Inport  Port=2
  wRW : Inport  Port=3
  SensorToBody (3x4) : Inport  Port=4
  IC3 : InitialCondition  Value=[wRW_init(1,1)*rw_Inertia; wRW_init(2,1)*rw_Inertia; wRW_init(3,1)*rw_Inertia;wRW_init(4,1)*rw_Inertia]
  IC4 : InitialCondition  Value=wRW_init
  Product1 : Product  Inputs=**  Multiplication=Matrix(*)  RndMeth=Zero
  Product3 : Product  Inputs=**  Multiplication=Matrix(*)  RndMeth=Zero
  Product4 : Product  Inputs=**  Multiplication=Matrix(*)  RndMeth=Zero
  Reshape{1..4,10..11} (6 alike) : Reshape  OutputDimensionality=Column vector (2-D)
  Hrw_dot : Outport  VectorParamsAs1DForOutWhenUnconnected=off
  w_RW_B : Outport  Port=2  VectorParamsAs1DForOutWhenUnconnected=off
  Hrw_B : Outport  Port=3  VectorParamsAs1DForOutWhenUnconnected=off
  wires:
  SensorToBody (3x4)/1 -> Product3/1, Product1/1, Product4/1  "Sensor To Body Frame"
  Product4/1 -> Reshape4/1
  Reshape1/1 -> Hrw_dot/1
  Reshape4/1 -> Hrw_B/1
  IC3/1 -> Product4/2
  IC4/1 -> Product1/2
  Product1/1 -> Reshape3/1
  Hrw/1 -> Reshape10/1
  Reshape10/1 -> IC3/1
  Reshape2/1 -> IC4/1
  wRW/1 -> Reshape2/1
  Reshape3/1 -> w_RW_B/1
  Reshape11/1 -> Product3/2
  Hrw_dot_1/1 -> Reshape11/1
  Product3/1 -> Reshape1/1

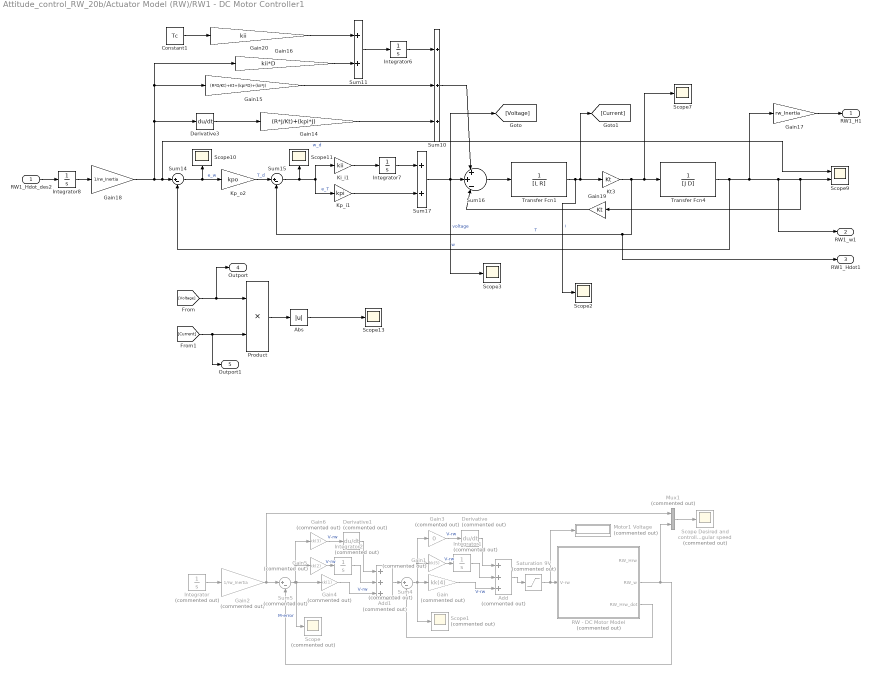
== system Attitude_control_RW_20b/Actuator Model (RW)/RW1 - DC Motor Controller1 ==
  RW1_Hdot_des2 : Inport
  Abs : Abs  SaturateOnIntegerOverflow=off
  Add : Sum  Commented=on  Inputs=+++
  Add1 : Sum  Commented=on  Inputs=+++
  Constant1 : Constant  Value=Tc
  Derivative : Derivative  Commented=on
  Derivative1 : Derivative  Commented=on
  Derivative3 : Derivative
  Gain : Gain  Commented=on  Gain=kk(4)
  Gain1 : Gain  Commented=on  Gain=kk(5)
  Gain14 : Gain  Gain=(R*J/Kt)+(kpi*J)
  Gain15 : Gain  Gain=(R*D/Kt)+Kt+(kpi*D)+(kii*J)
  Gain16 : Gain  Gain=kii*D
  Gain17 : Gain  Gain=rw_Inertia
  Gain18 : Gain  Gain=1/rw_Inertia
  Gain19 : Gain  Gain=Kt
  Gain2 : Gain  Commented=on  Gain=1/rw_Inertia
  Gain20 : Gain  Gain=kii
  Gain3 : Gain  Commented=on  Gain=0
  Gain4 : Gain  Commented=on  Gain=kk(1)
  Gain5 : Gain  Commented=on  Gain=kk(2)
  Gain6 : Gain  Commented=on  Gain=kk(3)
  Integrator : Integrator  Commented=on
  Integrator1 : Integrator  Commented=on
  Integrator2 : Integrator  Commented=on
  Integrator6 : Integrator
  Integrator7 : Integrator
  Integrator8 : Integrator
  Ki_i1 : Gain  Gain=kii
  Kp_i1 : Gain  Gain=kpi
  Kp_o2 : Gain  Gain=kpo
  Kt3 : Gain  Gain=Kt
  Motor1 Voltage : Display  Commented=on
  Mux1 : Mux  Commented=on  Inputs=2
  Product : Product
  RW - DC Motor Model : Subsystem  Commented=on
  "Saturation 9V " : Saturate  Commented=on  UpperLimit=9  LowerLimit=-9
  Scope : Scope  Commented=on
  "Scope Desired and controlled RW-angular speed " : Scope  Commented=on
  Scope1 : Scope  Commented=on
  Scope{2..3,7,10..11,13} (6 alike) : Scope
  Scope9 : Scope  NumInputPorts=2
  Sum10 : Sum  Inputs=+++
  Sum11 : Sum
  Sum14 : Sum  Inputs=|+-
  Sum15 : Sum  Inputs=|+-
  Sum16 : Sum  Inputs=|+|+|-|
  Sum17 : Sum
  Sum4 : Sum  Commented=on  Inputs=|+-
  Sum5 : Sum  Commented=on  Inputs=|+-
  Transfer Fcn1 : TransferFcn  Denominator=[L R]
  Transfer Fcn4 : TransferFcn  Denominator=[J D]
  RW1_H1 : Outport  VectorParamsAs1DForOutWhenUnconnected=off
  RW1_w1 : Outport  Port=2  VectorParamsAs1DForOutWhenUnconnected=off
  RW1_Hdot1 : Outport  Port=3  VectorParamsAs1DForOutWhenUnconnected=off
  Outport : Outport  Port=4
  Outport1 : Outport  Port=5
  wires:
  Gain4/1 -> Add1/3  "V-rw"
  Gain6/1 -> Derivative1/1  "V-rw"
  Derivative1/1 -> Add1/1
  RW - DC Motor Model/3(RW_Hrw_dot) -> Sum4/2
  Add1/1 -> Sum4/1
  Gain1/1 -> Integrator1/1  "V-rw"
  "Saturation 9V "/1 -> Motor1 Voltage/1, RW - DC Motor Model/1(V-rw)
  Gain3/1 -> Derivative/1  "V-rw"
  Add/1 -> "Saturation 9V "/1
  Gain/1 -> Add/3  "V-rw"
  Integrator1/1 -> Add/2
  Sum5/1 -> Gain6/1, Gain5/1, Scope/1, Gain4/1  "M-error"
  Mux1/1 -> "Scope Desired and controlled RW-angular speed "/1
  Sum4/1 -> Gain/1, Gain1/1, Gain3/1, Scope1/1
  Gain5/1 -> Integrator2/1  "V-rw"
  RW - DC Motor Model/2(RW_w) -> Sum5/2, Mux1/2
  Derivative/1 -> Add/1
  Integrator/1 -> Gain2/1
  Integrator2/1 -> Add1/2
  Gain2/1 -> Mux1/1, Sum5/1
  Gain15/1 -> Sum10/2
  Gain20/1 -> Sum11/1
  Gain14/1 -> Sum10/3
  Sum11/1 -> Integrator6/1
  Ki_i1/1 -> Integrator7/1
  Transfer Fcn4/1 -> Sum14/2, RW1_w1/1, Scope9/2, Gain19/1, Gain17/1  "w"
  Transfer Fcn1/1 -> Scope2/1, [Current], Kt3/1  "i"
  Sum14/1 -> Scope10/1, Kp_o2/1  "e_w"
  Derivative3/1 -> Gain14/1
  Gain16/1 -> Sum11/2
  Integrator8/1 -> Gain18/1
  Kt3/1 -> Sum15/2, RW1_Hdot1/1, Scope7/1, Transfer Fcn4/1  "T"
  Kp_i1/1 -> Sum17/2
  Sum15/1 -> Ki_i1/1, Kp_i1/1, Scope11/1  "e_T"
  Gain17/1 -> RW1_H1/1
  Integrator7/1 -> Sum17/1
  Constant1/1 -> Gain20/1
  Sum10/1 -> Sum16/1
  Sum17/1 -> Scope3/1, [Voltage], Sum16/2  "voltage"
  Gain18/1 -> Gain16/1, Gain15/1, Derivative3/1, Scope9/1, Sum14/1  "w_d"
  Sum16/1 -> Transfer Fcn1/1
  Integrator6/1 -> Sum10/1
  RW1_Hdot_des2/1 -> Integrator8/1
  Kp_o2/1 -> Sum15/1  "T_d"
  Gain19/1 -> Sum16/3
  [Current] -> Outport1/1, Product/2
  Abs/1 -> Scope13/1
  Product/1 -> Abs/1
  [Voltage] -> Outport/1, Product/1

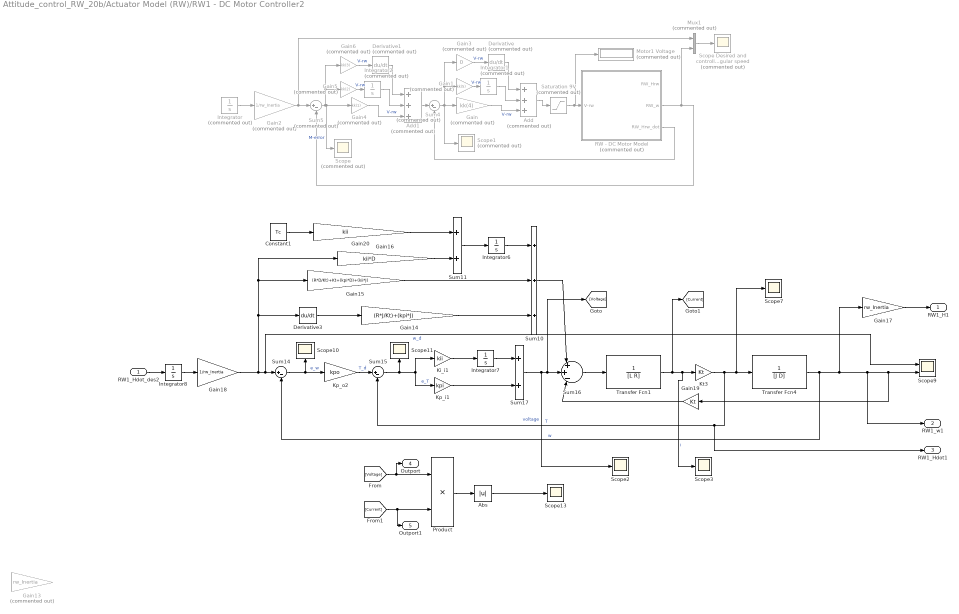
== system Attitude_control_RW_20b/Actuator Model (RW)/RW1 - DC Motor Controller2 ==
  RW1_Hdot_des2 : Inport
  Abs : Abs  SaturateOnIntegerOverflow=off
  Add : Sum  Commented=on  Inputs=+++
  Add1 : Sum  Commented=on  Inputs=+++
  Constant1 : Constant  Value=Tc
  Derivative : Derivative  Commented=on
  Derivative1 : Derivative  Commented=on
  Derivative3 : Derivative
  Gain : Gain  Commented=on  Gain=kk(4)
  Gain1 : Gain  Commented=on  Gain=kk(5)
  Gain13 : Gain  Commented=on  Gain=rw_Inertia
  Gain14 : Gain  Gain=(R*J/Kt)+(kpi*J)
  Gain15 : Gain  Gain=(R*D/Kt)+Kt+(kpi*D)+(kii*J)
  Gain16 : Gain  Gain=kii*D
  Gain17 : Gain  Gain=rw_Inertia
  Gain18 : Gain  Gain=1/rw_Inertia
  Gain19 : Gain  Gain=Kt
  Gain2 : Gain  Commented=on  Gain=1/rw_Inertia
  Gain20 : Gain  Gain=kii
  Gain3 : Gain  Commented=on  Gain=0
  Gain4 : Gain  Commented=on  Gain=kk(1)
  Gain5 : Gain  Commented=on  Gain=kk(2)
  Gain6 : Gain  Commented=on  Gain=kk(3)
  Integrator : Integrator  Commented=on
  Integrator1 : Integrator  Commented=on
  Integrator2 : Integrator  Commented=on
  Integrator6 : Integrator
  Integrator7 : Integrator
  Integrator8 : Integrator
  Ki_i1 : Gain  Gain=kii
  Kp_i1 : Gain  Gain=kpi
  Kp_o2 : Gain  Gain=kpo
  Kt3 : Gain  Gain=Kt
  Motor1 Voltage : Display  Commented=on
  Mux1 : Mux  Commented=on  Inputs=2
  Product : Product
  RW - DC Motor Model : Subsystem  Commented=on
  "Saturation 9V " : Saturate  Commented=on  UpperLimit=9  LowerLimit=-9
  Scope : Scope  Commented=on
  "Scope Desired and controlled RW-angular speed " : Scope  Commented=on
  Scope1 : Scope  Commented=on
  Scope{2..3,7,10..11,13} (6 alike) : Scope
  Scope9 : Scope  NumInputPorts=2
  Sum10 : Sum  Inputs=+++
  Sum11 : Sum
  Sum14 : Sum  Inputs=|+-
  Sum15 : Sum  Inputs=|+-
  Sum16 : Sum  Inputs=|+|+|-|
  Sum17 : Sum
  Sum4 : Sum  Commented=on  Inputs=|+-
  Sum5 : Sum  Commented=on  Inputs=|+-
  Transfer Fcn1 : TransferFcn  Denominator=[L R]
  Transfer Fcn4 : TransferFcn  Denominator=[J D]
  RW1_H1 : Outport  VectorParamsAs1DForOutWhenUnconnected=off
  RW1_w1 : Outport  Port=2  VectorParamsAs1DForOutWhenUnconnected=off
  RW1_Hdot1 : Outport  Port=3  VectorParamsAs1DForOutWhenUnconnected=off
  Outport : Outport  Port=4
  Outport1 : Outport  Port=5
  wires:
  Mux1/1 -> "Scope Desired and controlled RW-angular speed "/1
  Integrator2/1 -> Add1/2
  Derivative/1 -> Add/1
  RW - DC Motor Model/2(RW_w) -> Sum5/2, Mux1/2
  Integrator/1 -> Gain2/1
  Sum5/1 -> Gain6/1, Gain5/1, Scope/1, Gain4/1  "M-error"
  Sum4/1 -> Gain/1, Gain1/1, Gain3/1, Scope1/1
  Gain/1 -> Add/3  "V-rw"
  Integrator1/1 -> Add/2
  Gain1/1 -> Integrator1/1  "V-rw"
  Gain3/1 -> Derivative/1  "V-rw"
  Gain5/1 -> Integrator2/1  "V-rw"
  "Saturation 9V "/1 -> Motor1 Voltage/1, RW - DC Motor Model/1(V-rw)
  Add1/1 -> Sum4/1
  RW - DC Motor Model/3(RW_Hrw_dot) -> Sum4/2
  Derivative1/1 -> Add1/1
  Add/1 -> "Saturation 9V "/1
  Gain2/1 -> Mux1/1, Sum5/1
  Gain6/1 -> Derivative1/1  "V-rw"
  Gain4/1 -> Add1/3  "V-rw"
  Gain15/1 -> Sum10/2
  Gain20/1 -> Sum11/1
  Gain14/1 -> Sum10/3
  Sum11/1 -> Integrator6/1
  Ki_i1/1 -> Integrator7/1
  Transfer Fcn4/1 -> Sum14/2, RW1_w1/1, Scope9/2, Gain19/1, Gain17/1  "w"
  Transfer Fcn1/1 -> [Current], Scope3/1, Kt3/1  "i"
  Sum14/1 -> Scope10/1, Kp_o2/1  "e_w"
  Derivative3/1 -> Gain14/1
  Gain16/1 -> Sum11/2
  Integrator8/1 -> Gain18/1
  Kt3/1 -> Sum15/2, RW1_Hdot1/1, Scope7/1, Transfer Fcn4/1  "T"
  Kp_i1/1 -> Sum17/2
  Sum15/1 -> Ki_i1/1, Kp_i1/1, Scope11/1  "e_T"
  Gain17/1 -> RW1_H1/1
  Integrator7/1 -> Sum17/1
  Constant1/1 -> Gain20/1
  Sum10/1 -> Sum16/1
  Sum17/1 -> Scope2/1, [Voltage], Sum16/2  "voltage"
  Gain18/1 -> Gain16/1, Gain15/1, Derivative3/1, Scope9/1, Sum14/1  "w_d"
  Sum16/1 -> Transfer Fcn1/1
  Integrator6/1 -> Sum10/1
  RW1_Hdot_des2/1 -> Integrator8/1
  Kp_o2/1 -> Sum15/1  "T_d"
  Gain19/1 -> Sum16/3
  [Current] -> Outport1/1, Product/2
  Abs/1 -> Scope13/1
  Product/1 -> Abs/1
  [Voltage] -> Outport/1, Product/1

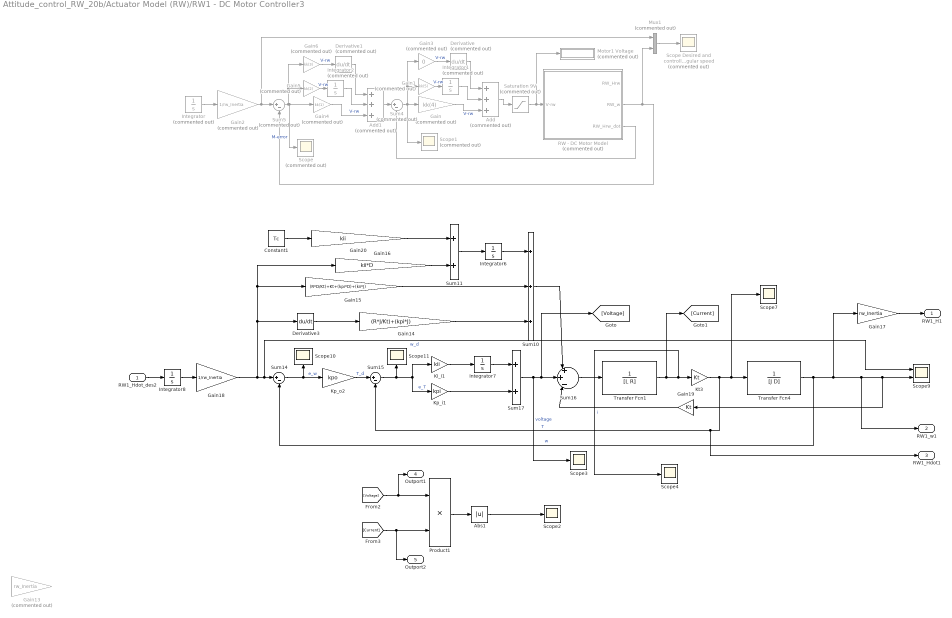
== system Attitude_control_RW_20b/Actuator Model (RW)/RW1 - DC Motor Controller3 ==
  RW1_Hdot_des2 : Inport
  Abs1 : Abs  SaturateOnIntegerOverflow=off
  Add : Sum  Commented=on  Inputs=+++
  Add1 : Sum  Commented=on  Inputs=+++
  Constant1 : Constant  Value=Tc
  Derivative : Derivative  Commented=on
  Derivative1 : Derivative  Commented=on
  Derivative3 : Derivative
  Gain : Gain  Commented=on  Gain=kk(4)
  Gain1 : Gain  Commented=on  Gain=kk(5)
  Gain13 : Gain  Commented=on  Gain=rw_Inertia
  Gain14 : Gain  Gain=(R*J/Kt)+(kpi*J)
  Gain15 : Gain  Gain=(R*D/Kt)+Kt+(kpi*D)+(kii*J)
  Gain16 : Gain  Gain=kii*D
  Gain17 : Gain  Gain=rw_Inertia
  Gain18 : Gain  Gain=1/rw_Inertia
  Gain19 : Gain  Gain=Kt
  Gain2 : Gain  Commented=on  Gain=1/rw_Inertia
  Gain20 : Gain  Gain=kii
  Gain3 : Gain  Commented=on  Gain=0
  Gain4 : Gain  Commented=on  Gain=kk(1)
  Gain5 : Gain  Commented=on  Gain=kk(2)
  Gain6 : Gain  Commented=on  Gain=kk(3)
  Integrator : Integrator  Commented=on
  Integrator1 : Integrator  Commented=on
  Integrator2 : Integrator  Commented=on
  Integrator6 : Integrator
  Integrator7 : Integrator
  Integrator8 : Integrator
  Ki_i1 : Gain  Gain=kii
  Kp_i1 : Gain  Gain=kpi
  Kp_o2 : Gain  Gain=kpo
  Kt3 : Gain  Gain=Kt
  Motor1 Voltage : Display  Commented=on
  Mux1 : Mux  Commented=on  Inputs=2
  Product1 : Product
  RW - DC Motor Model : Subsystem  Commented=on
  "Saturation 9V " : Saturate  Commented=on  UpperLimit=9  LowerLimit=-9
  Scope : Scope  Commented=on
  "Scope Desired and controlled RW-angular speed " : Scope  Commented=on
  Scope1 : Scope  Commented=on
  Scope{2..4,7,10..11} (6 alike) : Scope
  Scope9 : Scope  NumInputPorts=2
  Sum10 : Sum  Inputs=+++
  Sum11 : Sum
  Sum14 : Sum  Inputs=|+-
  Sum15 : Sum  Inputs=|+-
  Sum16 : Sum  Inputs=|+|+|-|
  Sum17 : Sum
  Sum4 : Sum  Commented=on  Inputs=|+-
  Sum5 : Sum  Commented=on  Inputs=|+-
  Transfer Fcn1 : TransferFcn  Denominator=[L R]
  Transfer Fcn4 : TransferFcn  Denominator=[J D]
  RW1_H1 : Outport  VectorParamsAs1DForOutWhenUnconnected=off
  RW1_w1 : Outport  Port=2  VectorParamsAs1DForOutWhenUnconnected=off
  RW1_Hdot1 : Outport  Port=3  VectorParamsAs1DForOutWhenUnconnected=off
  Outport1 : Outport  Port=4
  Outport2 : Outport  Port=5
  wires:
  Mux1/1 -> "Scope Desired and controlled RW-angular speed "/1
  Integrator2/1 -> Add1/2
  Derivative/1 -> Add/1
  RW - DC Motor Model/2(RW_w) -> Sum5/2, Mux1/2
  Integrator/1 -> Gain2/1
  Sum5/1 -> Gain6/1, Gain5/1, Scope/1, Gain4/1  "M-error"
  Sum4/1 -> Gain/1, Gain1/1, Gain3/1, Scope1/1
  Gain/1 -> Add/3  "V-rw"
  Integrator1/1 -> Add/2
  Gain1/1 -> Integrator1/1  "V-rw"
  Gain3/1 -> Derivative/1  "V-rw"
  Gain5/1 -> Integrator2/1  "V-rw"
  "Saturation 9V "/1 -> Motor1 Voltage/1, RW - DC Motor Model/1(V-rw)
  Add1/1 -> Sum4/1
  RW - DC Motor Model/3(RW_Hrw_dot) -> Sum4/2
  Derivative1/1 -> Add1/1
  Add/1 -> "Saturation 9V "/1
  Gain2/1 -> Mux1/1, Sum5/1
  Gain6/1 -> Derivative1/1  "V-rw"
  Gain4/1 -> Add1/3  "V-rw"
  Gain15/1 -> Sum10/2
  Gain20/1 -> Sum11/1
  Gain14/1 -> Sum10/3
  Sum11/1 -> Integrator6/1
  Ki_i1/1 -> Integrator7/1
  Transfer Fcn4/1 -> Sum14/2, RW1_w1/1, Scope9/2, Gain19/1, Gain17/1  "w"
  Transfer Fcn1/1 -> [Current], Scope4/1, Kt3/1  "i"
  Sum14/1 -> Scope10/1, Kp_o2/1  "e_w"
  Derivative3/1 -> Gain14/1
  Gain16/1 -> Sum11/2
  Integrator8/1 -> Gain18/1
  Kt3/1 -> Sum15/2, RW1_Hdot1/1, Scope7/1, Transfer Fcn4/1  "T"
  Kp_i1/1 -> Sum17/2
  Sum15/1 -> Ki_i1/1, Kp_i1/1, Scope11/1  "e_T"
  Gain17/1 -> RW1_H1/1
  Integrator7/1 -> Sum17/1
  Constant1/1 -> Gain20/1
  Sum10/1 -> Sum16/1
  Sum17/1 -> Scope3/1, [Voltage], Sum16/2  "voltage"
  Gain18/1 -> Gain16/1, Gain15/1, Derivative3/1, Scope9/1, Sum14/1  "w_d"
  Sum16/1 -> Transfer Fcn1/1
  Integrator6/1 -> Sum10/1
  RW1_Hdot_des2/1 -> Integrator8/1
  Kp_o2/1 -> Sum15/1  "T_d"
  Gain19/1 -> Sum16/3
  [Current] -> Outport2/1, Product1/2
  Abs1/1 -> Scope2/1
  Product1/1 -> Abs1/1
  [Voltage] -> Outport1/1, Product1/1

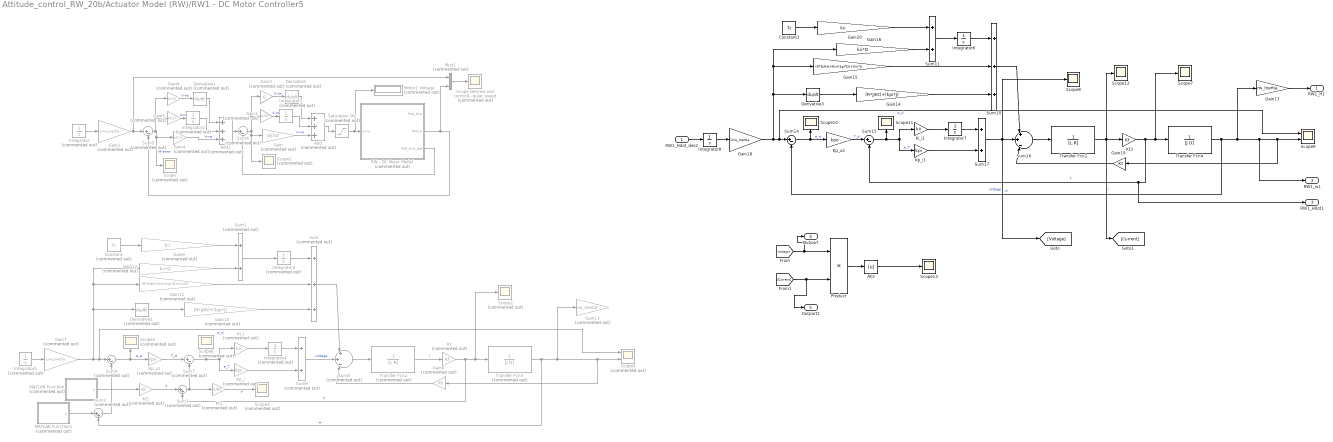
== system Attitude_control_RW_20b/Actuator Model (RW)/RW1 - DC Motor Controller5 ==
  RW1_Hdot_des2 : Inport
  Abs : Abs  SaturateOnIntegerOverflow=off
  Add : Sum  Commented=on  Inputs=+++
  Add1 : Sum  Commented=on  Inputs=+++
  Constant : Constant  Commented=on  Value=Tc
  Constant1 : Constant  Value=Tc
  Derivative : Derivative  Commented=on
  Derivative1 : Derivative  Commented=on
  Derivative2 : Derivative  Commented=on
  Derivative3 : Derivative
  Gain : Gain  Commented=on  Gain=kk(4)
  Gain1 : Gain  Commented=on  Gain=kk(5)
  Gain10 : Gain  Commented=on  Gain=(R*J/Kt)+(kpi*J)
  Gain11 : Gain  Commented=on  Gain=(R*D/Kt)+Kt+(kpi*D)+(kii*J)
  Gain12 : Gain  Commented=on  Gain=kii*D
  Gain13 : Gain  Commented=on  Gain=rw_Inertia
  Gain14 : Gain  Gain=(R*J/Kt)+(kpi*J)
  Gain15 : Gain  Gain=(R*D/Kt)+Kt+(kpi*D)+(kii*J)
  Gain16 : Gain  Gain=kii*D
  Gain17 : Gain  Gain=rw_Inertia
  Gain18 : Gain  Gain=1/rw_Inertia
  Gain19 : Gain  Gain=Kt
  Gain2 : Gain  Commented=on  Gain=1/rw_Inertia
  Gain20 : Gain  Gain=kii
  Gain3 : Gain  Commented=on  Gain=0
  Gain4 : Gain  Commented=on  Gain=kk(1)
  Gain5 : Gain  Commented=on  Gain=kk(2)
  Gain6 : Gain  Commented=on  Gain=kk(3)
  Gain7 : Gain  Commented=on  Gain=1/rw_Inertia
  Gain8 : Gain  Commented=on  Gain=Kt
  Gain9 : Gain  Commented=on  Gain=kii
  Integrator{,1..5} (6 alike) : Integrator  Commented=on
  Integrator6 : Integrator
  Integrator7 : Integrator
  Integrator8 : Integrator
  Ki_i : Gain  Commented=on  Gain=kii
  Ki_i1 : Gain  Gain=kii
  Kp_i : Gain  Commented=on  Gain=kpi
  Kp_i1 : Gain  Gain=kpi
  Kp_o1 : Gain  Commented=on  Gain=kpo
  Kp_o2 : Gain  Gain=kpo
  Kt : Gain  Commented=on  Gain=Kt
  Kt1 : Gain  Commented=on  Gain=Kt
  Kt2 : Gain  Commented=on  Gain=1/Kt
  Kt3 : Gain  Gain=Kt
  MATLAB Function : MATLAB Function  Commented=on  TreatAsAtomicUnit=on
  MATLAB Function1 : MATLAB Function  Commented=on  TreatAsAtomicUnit=on
  Motor1 Voltage : Display  Commented=on
  Mux1 : Mux  Commented=on  Inputs=2
  Product : Product
  RW - DC Motor Model : Subsystem  Commented=on
  "Saturation 9V " : Saturate  Commented=on  UpperLimit=9  LowerLimit=-9
  Scope{,1..3,5..6} (6 alike) : Scope  Commented=on
  "Scope Desired and controlled RW-angular speed " : Scope  Commented=on
  Scope{7..8,10..13} (6 alike) : Scope
  Scope4 : Scope  Commented=on  NumInputPorts=2
  Scope9 : Scope  NumInputPorts=2
  Sum : Sum  Commented=on  Inputs=+++
  Sum1 : Sum  Commented=on
  Sum10 : Sum  Inputs=+++
  Sum11 : Sum
  Sum14 : Sum  Inputs=|+-
  Sum15 : Sum  Inputs=|+-
  Sum16 : Sum  Inputs=|+|+|-|
  Sum17 : Sum
  Sum2 : Sum  Commented=on  Inputs=|++
  Sum3 : Sum  Commented=on  Inputs=|++
  Sum{4..7} (4 alike) : Sum  Commented=on  Inputs=|+-
  Sum8 : Sum  Commented=on  Inputs=|+|+|-|
  Sum9 : Sum  Commented=on
  Transfer Fcn1 : TransferFcn  Denominator=[L R]
  Transfer Fcn2 : TransferFcn  Commented=on  Denominator=[L R]
  Transfer Fcn3 : TransferFcn  Commented=on  Denominator=[J D]
  Transfer Fcn4 : TransferFcn  Denominator=[J D]
  RW1_H1 : Outport  VectorParamsAs1DForOutWhenUnconnected=off
  RW1_w1 : Outport  Port=2  VectorParamsAs1DForOutWhenUnconnected=off
  RW1_Hdot1 : Outport  Port=3  VectorParamsAs1DForOutWhenUnconnected=off
  Outport : Outport  Port=4
  Outport1 : Outport  Port=5
  wires:
  Integrator/1 -> Gain2/1
  Sum4/1 -> Gain/1, Scope1/1, Gain1/1, Gain3/1
  RW - DC Motor Model/2(RW_w) -> Sum5/2, Mux1/2
  Add1/1 -> Sum4/1
  Sum5/1 -> Gain6/1, Gain5/1, Scope/1, Gain4/1  "M-error"
  Mux1/1 -> "Scope Desired and controlled RW-angular speed "/1
  Gain2/1 -> Mux1/1, Sum5/1
  "Saturation 9V "/1 -> Motor1 Voltage/1, RW - DC Motor Model/1(V-rw)
  RW - DC Motor Model/3(RW_Hrw_dot) -> Sum4/2
  Add/1 -> "Saturation 9V "/1
  Gain1/1 -> Integrator1/1  "V-rw"
  Gain/1 -> Add/3  "V-rw"
  Integrator1/1 -> Add/2
  Gain3/1 -> Derivative/1  "V-rw"
  Derivative/1 -> Add/1
  Derivative1/1 -> Add1/1
  Gain6/1 -> Derivative1/1  "V-rw"
  Integrator2/1 -> Add1/2
  Gain4/1 -> Add1/3  "V-rw"
  Gain5/1 -> Integrator2/1  "V-rw"
  Kt2/1 -> Scope3/1  "T"
  MATLAB Function1/1(y) -> Sum2/1
  Integrator4/1 -> Sum9/1
  Sum9/1 -> Sum8/2  "voltage"
  Sum2/1 -> Sum6/2
  Kt1/1 -> Sum3/1  "T"
  Sum/1 -> Sum8/1
  MATLAB Function/1(y) -> Kt1/1
  Sum8/1 -> Transfer Fcn2/1
  Integrator3/1 -> Sum/1
  Constant/1 -> Gain9/1
  Sum1/1 -> Integrator3/1
  Gain10/1 -> Sum/3
  Sum3/1 -> Kt2/1, Sum7/2
  Ki_i/1 -> Integrator4/1
  Gain11/1 -> Sum/2
  Derivative2/1 -> Gain10/1
  Gain9/1 -> Sum1/1
  Gain7/1 -> Derivative2/1, Gain11/1, Gain12/1, Scope4/1, Sum6/1  "w_d"
  Transfer Fcn3/1 -> Scope4/2, Gain8/1, Gain13/1, Sum2/2  "w"
  Sum6/1 -> Kp_o1/1, Scope5/1  "e_w"
  Kp_o1/1 -> Sum7/1  "T_d"
  Sum7/1 -> Ki_i/1, Kp_i/1, Scope6/1  "e_T"
  Gain12/1 -> Sum1/2
  Transfer Fcn2/1 -> Kt/1  "i"
  Kp_i/1 -> Sum9/2
  Kt/1 -> Sum3/2, Scope2/1, Transfer Fcn3/1  "T"
  Gain8/1 -> Sum8/3
  Integrator5/1 -> Gain7/1
  RW1_Hdot_des2/1 -> Integrator8/1
  Gain19/1 -> Sum16/3
  Kt3/1 -> Sum15/2, RW1_Hdot1/1, Scope7/1, Transfer Fcn4/1  "T"
  Integrator8/1 -> Gain18/1
  Kp_i1/1 -> Sum17/2
  Gain16/1 -> Sum11/2
  Sum15/1 -> Ki_i1/1, Kp_i1/1, Scope11/1  "e_T"
  Sum14/1 -> Scope10/1, Kp_o2/1  "e_w"
  Transfer Fcn4/1 -> Sum14/2, RW1_w1/1, Scope9/2, Gain19/1, Gain17/1  "w"
  Transfer Fcn1/1 -> [Current], Scope12/1, Kt3/1  "i"
  Gain18/1 -> Gain16/1, Gain15/1, Derivative3/1, Scope9/1, Sum14/1  "w_d"
  Gain20/1 -> Sum11/1
  Derivative3/1 -> Gain14/1
  Gain15/1 -> Sum10/2
  Gain14/1 -> Sum10/3
  Ki_i1/1 -> Integrator7/1
  Sum11/1 -> Integrator6/1
  Kp_o2/1 -> Sum15/1  "T_d"
  Integrator6/1 -> Sum10/1
  Sum16/1 -> Transfer Fcn1/1
  Sum10/1 -> Sum16/1
  Sum17/1 -> Scope8/1, [Voltage], Sum16/2  "voltage"
  Constant1/1 -> Gain20/1
  Gain17/1 -> RW1_H1/1
  Integrator7/1 -> Sum17/1
  [Voltage] -> Outport/1, Product/1
  [Current] -> Outport1/1, Product/2
  Product/1 -> Abs/1
  Abs/1 -> Scope13/1

== system Attitude_control_RW_20b/Controller/Subsystem ==
  Euler Angles : Inport
  Degrees to Radians1 : simulink_extras/Transformations/Degrees to Radians
  Direction Cosine Matrix to Quaternions : sharedtransform/Direction Cosine Matrix  to Quaternions  aMode=0  action=None  tolerance=eps(2)
      settings: SourceProductBaseCode=AE,PW,DR,MT,VE
  Rotation Angles to Direction Cosine Matrix : sharedtransform/Rotation Angles to Direction Cosine Matrix  rotationOrder=ZYX  aMode=aMode
      settings: SourceProductBaseCode=AE,PW,DR,MT,VE
  Subsystem1 : Subsystem
  qRef : Outport  VectorParamsAs1DForOutWhenUnconnected=off
  wires:
  Euler Angles/1 -> Degrees to Radians1/1
  Degrees to Radians1/1 -> Rotation Angles to Direction Cosine Matrix/1
  Rotation Angles to Direction Cosine Matrix/1 -> Direction Cosine Matrix to Quaternions/1
  Direction Cosine Matrix to Quaternions/1 -> Subsystem1/1(q0,q1,q2,q3)
  Subsystem1/1(q1,q2,q3,q4) -> qRef/1
